simulink model "Simulink_NLS"  (R2024a)
settings: Solver=VariableStepAuto  StartTime=0.0  StopTime=0.04  RelTol=1e-3
libraries: simulink_extras x1, hdlsllib x1
settings Model: Creator=divya  LastModifiedBy=h2kjp

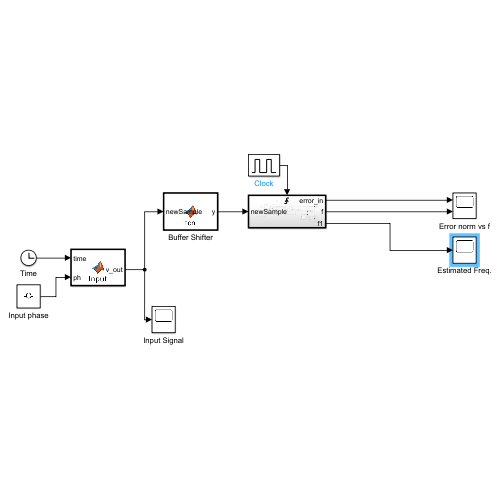
[thumbnail: Simulink's stored preview of the top-level diagram]
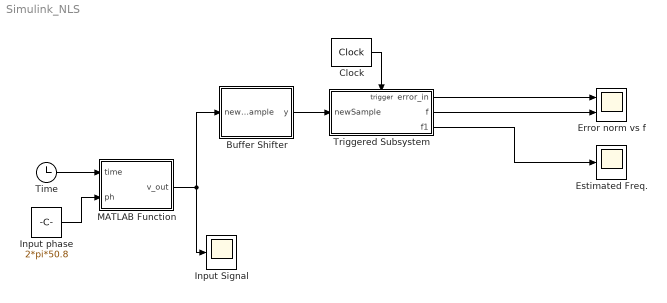
== system Simulink_NLS ==
  Buffer Shifter : MATLAB Function  TreatAsAtomicUnit=on  SystemSampleTime=0.000625
  Clock : simulink_extras/Flip Flops/Clock  period=0.625e-6
  Error norm vs f : Scope  NumInputPorts=2
  Estimated Freq. : Scope
  Input Signal : Scope
  Input phase : Constant  Value=2*pi*50.8
  MATLAB Function : MATLAB Function  TreatAsAtomicUnit=on  SystemSampleTime=0.000005
  Time : Clock
  Triggered Subsystem : Subsystem  TreatAsAtomicUnit=on
  wires:
  Clock/1 -> Triggered Subsystem/Trigger
  Triggered Subsystem/1(error_in) -> Error norm vs f/1
  Triggered Subsystem/2(f) -> Error norm vs f/2
  Buffer Shifter/1(y) -> Triggered Subsystem/1(newSample)
  Triggered Subsystem/3(f1) -> Estimated Freq./1
  Time/1 -> MATLAB Function/1(time)
  Input phase/1 -> MATLAB Function/2(ph)
  MATLAB Function/1(v_out) -> Input Signal/1, Buffer Shifter/1(newSample)

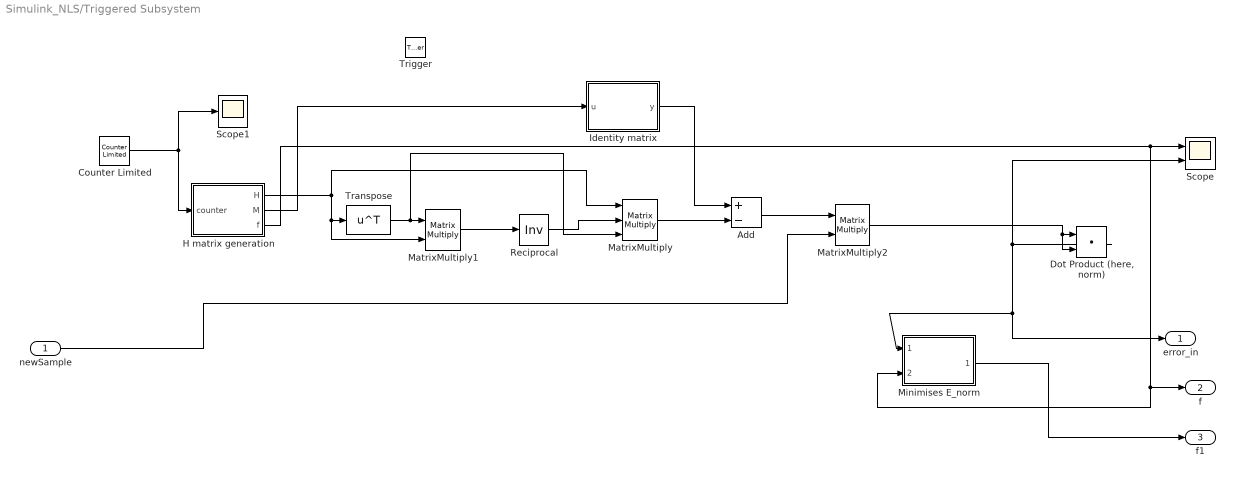
== system Simulink_NLS/Triggered Subsystem ==
  newSample : Inport
  Trigger : TriggerPort  VariantControl=(inherit)
  Add : Sum  Inputs=+-
  Counter Limited : hdlsllib/Sources/Counter Limited  uplimit=30  tsamp=-1
  "Dot Product (here, norm)" : DotProduct  OutDataTypeStr=Inherit: Inherit via internal rule
  H matrix generation : MATLAB Function  TreatAsAtomicUnit=on
  Identity matrix : MATLAB Function  TreatAsAtomicUnit=on
  MatrixMultiply : Product  Inputs=3  Multiplication=Matrix(*)
  MatrixMultiply1 : Product  Multiplication=Matrix(*)
  MatrixMultiply2 : Product  Multiplication=Matrix(*)
  Minimises E_norm : MATLAB Function  TreatAsAtomicUnit=on
  Reciprocal : Product  Inputs=/  Multiplication=Matrix(*)  RndMeth=Zero  SaturateOnIntegerOverflow=on
  Scope : Scope  NumInputPorts=2
  Scope1 : Scope
  Transpose : Math  Operator=transpose  SignedPower=on  RndMeth=Zero
  error_in : Outport
  f : Outport  Port=2
  f1 : Outport  Port=3
  wires:
  MatrixMultiply/1 -> Add/2
  Identity matrix/1(y) -> Add/1
  MatrixMultiply1/1 -> Reciprocal/1
  Transpose/1 -> MatrixMultiply/3, MatrixMultiply1/1
  Add/1 -> MatrixMultiply2/1
  H matrix generation/1(H) -> MatrixMultiply/1, MatrixMultiply1/2, Transpose/1
  Reciprocal/1 -> MatrixMultiply/2
  Counter Limited/1 -> H matrix generation/1(counter), Scope1/1
  H matrix generation/2(M) -> Identity matrix/1(u)
  "Dot Product (here, norm)"/1 -> error_in/1, Minimises E_norm/1(error_in), Scope/2
  MatrixMultiply2/1 -> "Dot Product (here, norm)"/2, "Dot Product (here, norm)"/1
  newSample/1 -> MatrixMultiply2/2
  H matrix generation/3(f) -> Scope/1, Minimises E_norm/2(freq_in), f/1
  Minimises E_norm/1(freq_best) -> f1/1

== matlab function Simulink_NLS/Buffer Shifter ==
  data: y output size=16,1; newSample input
function y = fcn(newSample)
%#codegen

% Define window size for the buffer (16 samples ~ 10 ms at 1.6 kHz)
N_window = 16;

% Declare persistent variables for the sample buffer and sample counter
persistent buffer sampleCount

% Initialize persistent variables if empty
if isempty(sampleCount)
    % Ts = 1/1600;            % The sampling period (not currently used in this snippet)
    buffer = zeros(N_window, 1); 
    sampleCount = 0;
    
    % The following variables are not used yet, so you can comment them out or keep them:
    % f_prev = 50;                     
    % allowed_harmonics = [1, 5, 7, 11, 13]; 
end

% Accumulate samples until the buffer is full; then use a sliding window
if sampleCount < N_window
    sampleCount = sampleCount + 1;
    buffer(sampleCount) = newSample;
    
    % Since the buffer is not yet full, define y as something
    % e.g. zeros(N_window,1) or the partial buffer
    % For code generation, y must be defined in every branch
    y = zeros(N_window,1);  % or y = buffer if you prefer
    return;
else
    % Slide the window by one sample and append the new sample
    buffer(1:end-1) = buffer(2:end);
    buffer(end) = newSample;
end

% Now the buffer is full, we can set y to be the entire buffer (or something else)
y = buffer;  % <--- Replaced invalid // comment with a valid MATLAB comment

== matlab function Simulink_NLS/MATLAB Function ==
  data: time input; v_out output; ph input
function v_out = Input(time, ph)
omega0=ph;
%#codegen
% v(t) = sin(omega0 * t)
%      + 0.0856*sin(5*omega0*t)
%      + 0.0428*sin(7*omega0*t)
%      + 0.0306*sin(11*omega0*t)
%      + 0.0183*sin(13*omega0*t)

    v_out = ...
        sin(omega0 * time) + ...
        0.0856 * sin(5 * omega0 * time) + ...
        0.0428 * sin(7 * omega0 * time) + ...
        0.0306 * sin(11 * omega0 * time) + ...
        0.0183 * sin(13 * omega0 * time);
end

== matlab function Simulink_NLS/Triggered Subsystem/H matrix generation ==
  data: counter input; H output size=16,10; M output; f output
function [H,M,f]= generateHMatrix(counter)
    % Define the sampling frequency and window size
    nh=13;
    window_size_ms=10;
    Fs = 1600; % Sampling frequency (1.6 kHz)
    Ts = 1 / Fs; % Sampling period
    N_window = round(window_size_ms / 1000 * Fs); % Number of samples in the window (10ms)
    t_window = (0:N_window-1) * Ts; % Time vector for the window
    M=N_window;
    % Define the frequency range for counter (48.5 Hz to 51.5 Hz, increasing by 0.1 Hz per counter step)
    f_start = 48.5; % Start frequency (Hz)
    f_step = 0.1;   % Step size (Hz)
    f_current = double(f_start + double(counter) * f_step); % Calculate current frequency based on counter
    f=double(f_current);
    % Initialize matrix H (size N_window x 2 * nh)
    H = zeros(N_window, 2 * 5);
    ah = [1.0, 5.0, 7.0, 11.0, 13.0];
    % Generate the H matrix (sin and cos components for each harmonic)
    % --- Only change the loop portion ---
for h = 1:5
    % Fill columns 1..5 with cosines
    H(:, h) = cos(2 * pi * f_current * ah(h) * t_window);
    % Fill columns 6..10 with sines
    H(:, 5 + h) = sin(2 * pi * f_current * ah(h) * t_window);
end

end

== matlab function Simulink_NLS/Triggered Subsystem/Identity matrix ==
  data: u input; y output size=16,16
function y = fcn(u)
%#codegen

y = eye(16,16);

== matlab function Simulink_NLS/Triggered Subsystem/Minimises E_norm ==
  data: error_in input; freq_best output; freq_in input
function freq_best = PickMinFreq(error_in, freq_in)
%#codegen
% This function takes as inputs:
%   error_in: the error computed for the current candidate frequency
%   freq_in : the current candidate frequency (e.g., sweeping from 48.5 to 51.5 Hz)
%
% It outputs:
%   freq_best: the best frequency (with minimum error) from the previous complete sweep.
%
% The output is held constant for the entire sample window and only updated
% when a new sweep is detected (i.e. when freq_in resets from a high value back
% to the starting frequency).

    persistent bestError bestFreq currentBest lastFreq initDone
    if isempty(initDone)
        % Initialization on first call
        bestError   = inf;
        bestFreq    = freq_in;
        currentBest = freq_in;
        lastFreq    = freq_in;
        initDone    = true;
    end

    % Detect wrap-around: new sweep when current candidate is lower than the previous one.
    if freq_in < lastFreq
        % A new sweep has started.
        % Finalize the best frequency from the previous sweep:
        currentBest = bestFreq;
        
        % Reset for the new sweep with the current candidate.
        bestError = error_in;
        bestFreq  = freq_in;
    else
        % In the same sweep: update best candidate if the current error is lower.
        if error_in < bestError
            bestError = error_in;
            bestFreq  = freq_in;
        end
    end

    % Update last frequency for next call.
    lastFreq = freq_in;
    
    % Output the best frequency from the previous sweep.
    freq_best = currentBest;
end
